simulink model "MultirotorSimPx4v1_8TuningRateCont"  (R2018b)
settings: Solver=VariableStepAuto  StartTime=0.0  StopTime=Simulation.T_END  MaxStep=Simulation.TS_MAX  RelTol=1e-3  EnableMultiTasking=on
PreLoadFcn:
  | % InitializeParameters;
undefined symbols (not defined in the file): DiscIntNeverNeededParam, Initial, Simulation, Uav, Wind
libraries: QuaternionLibrary x10, simulink x3, simulink_extras x2
(part 1 of 2)
settings Model: PauseTimes=0.99  Creator=jban039  LastModifiedBy=jban039
settings DataIOCC: Decimation=10  ExternalInput=getinputstruct(op1(2))  InitialState=getstatestruct(op)  SaveFormat=StructureWithTime  ReturnWorkspaceOutputs=on  OutputTimes=Simulation.T_OUT
settings OptimizationCC: LifeSpan=inf
settings DebuggingCC: ReadBeforeWriteMsg=DisableAll  WriteAfterWriteMsg=DisableAll  WriteAfterReadMsg=DisableAll  MultiTaskDSMMsg=none  UnconnectedLineMsg=none  AllowSymbolicDim=off  SFUnexpectedBacktrackingDiag=warning  SFNoUnconditionalDefaultTransitionDiag=warning  SFExecutionAtInitializationDiag=none
settings ModelReferenceCC: UpdateModelReferenceTargets=IfOutOfDate  ModelReferenceMinAlgLoopOccurrences=on  PropagateSignalLabelsOutOfModel=off
settings SFSimCC: SFSimEcho=off  SimUseLocalCustomCode=off
settings RTWCC: RTWUseLocalCustomCode=off
settings CodeAppCC: StateflowObjectComments=on
settings GRTTargetCC: TargetLangStandard=C89/C90 (ANSI)
settings ConfigComp: CovMetricSettings=dw  CovHtmlReporting=on  CovSaveCumulativeToWorkspaceVar=on  CovSaveSingleToWorkspaceVar=on  CovExternalEMLEnable=off

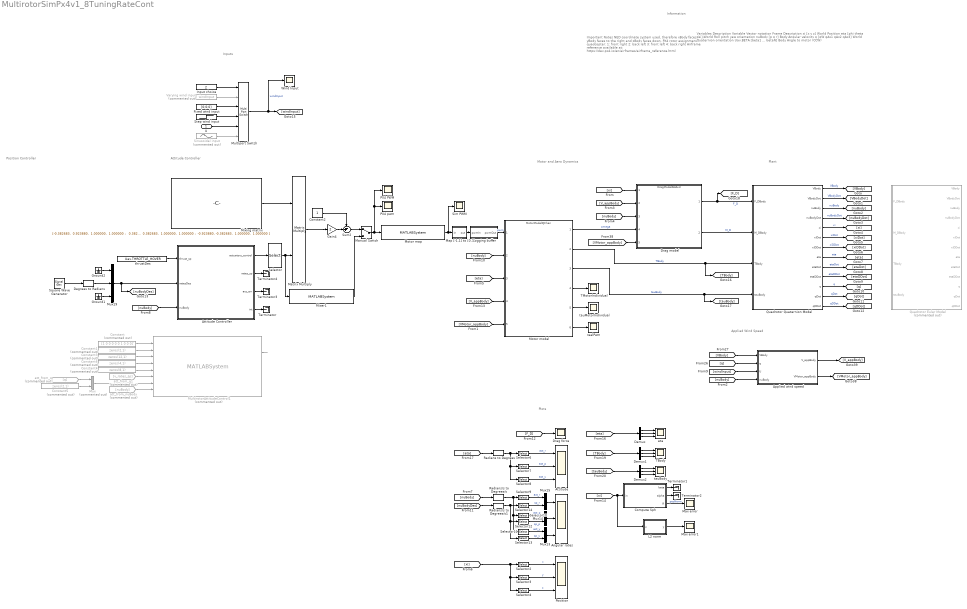
== system MultirotorSimPx4v1_8TuningRateCont ==
  note: Plots
  note: Inputs
  note: Motor and Aero Dynamics
  note: Plant
  note: Attitude Controller
  note: Position Controller
  note: Applied Wind Speed
  note: Important Notes
      |
      | NED coordinate system used, therefore xBody faces forward, yBody faces to the right and zBody faces down.
      | PX4 rotor assignment for quadcopter:
      | 1: front right
      | 2: back left
      | 3: front left
      | 4: back right
      | Airframe reference available at:
      | https://dev.px4.io/en/airframes/airframe_reference.html
  note: Variables Description
      |
      | Variable
      | Vector notation
      | Frame
      | Description
      |
      | xi
      | [x y z]
      | World
      | Position
      |
      | eta
      | [phi theta psi]
      | World
      | Roll pitch yaw orientation
      |
      | nuBody
      | [p q r]
      | Body
      | Angular velocity
      |
      | q
      | [qW qAx1 qAx2 qAx3]
      | World
      | Quaternion orientation
      |
      | Uav.BETA
      | [beta1 ... betaN]
      | Body
      | Angle to motor (CCW)
  note: Information
  U : Inport  PortDimensions=3
  Angular rates : Scope  NumInputPorts=3
  Applied wind speed : Subsystem
  Attitude : Scope  NumInputPorts=3
  Attitude Controller : Subsystem
  Compute Sph : MATLAB Function  TreatAsAtomicUnit=on
  Constant : Constant  Commented=on  Value=[1 0 0 0 0 0 1 0 0 0]'
  Constant1 : Constant  Commented=on  Value=zeros(2,1)
  Constant2 : Constant
  Constant3 : Constant  Commented=on  Value=zeros(12,1)
  Constant4 : Constant  Commented=on  Value=zeros(8,1)
  Constant5 : Constant  Commented=on  Value=zeros(2,1)
  Constant6 : Constant  Commented=on  Value=zeros(4,1)
  Degrees to Radians : simulink_extras/Transformations/Degrees to Radians
  Demux : Demux  Outputs=3
  Demux1 : Demux  Outputs=3
  Demux2 : Demux  Outputs=3
  Drag force : Scope
  Drag model : ModelReference  ModelNameDialog=DragModelAIAAv3  SimulationMode=Normal  ModelReferenceVersion=1.368
  Fixed wind input : Constant  Value=[0;0;0]
  Gain4 : Gain  Gain=2
  Ground1 : Ground
  Ground2 : Ground
  Input choice : Constant  Value=2
  L2 norm : MATLAB Function  TreatAsAtomicUnit=on
  Logging buffer : Subsystem
  Manual Switch : ManualSwitch
  Map [-1,1] to [0,1] : Subsystem
  Matrix Multiply : Product  Multiplication=Matrix(*)
  Max error : Scope
  Max error1 : Scope
  Mixer1 : MATLABSystem  System=MultirotorMixer  airframeConfig=6  useHorThrust=0  outputSatStatus=0  SimulateUsing=Code generation
      mask Type: MultirotorMixer
      mask Display:
      | disp(['MULTIROTOR' char(10) 'MIXER' char(10) 'octa_xneg']);
      | port_label('input',1,'actuatorsControl');
      | port_label('output',1,'px4PWM');
  Mixing matrix : Constant  Value=|
      | [-0.382683,  0.923880,  1.000000,  1.000000 ;
      |   0.382683, -0.923880,  1.000000,  1.000000 ;
      |  -0.923880,  0.382683, -1.000000,  1.000000 ;
      |  -0.382683, -0.923880, -1.000000,  1.000000 ;
      |   0.382683,  0.923880, -1.000000,  1.000000 ;
      |   0.923880, -0.382683, -1.000000,  1.000000 ;
      |   0.923880,  0.382683,  1.000000,  1.000000 ;
      |  -0.923880, -0.382683,  1.000000,  1.000000 ]
  Motor map : MATLABSystem  System=MotorMap  airframeConfig=5  SimulateUsing=Code generation
      mask Type: MotorMap
      mask Display:
      | disp(['MOTOR' char(10) 'MAP' char(10) 'octa_x']);
      | port_label('input',1,'px4PWM');
      | port_label('output',1,'simPWM');
  Motor model : ModelReference  ModelNameDialog=MotorModelZJChen  SimulationMode=Normal  ModelReferenceVersion=1.421
  Multiport Switch : MultiPortSwitch  Inputs=5
  MultirotorAttitudeControl1 : MATLABSystem  Commented=on  System=MulticopterAttitudeControl  acro_expo_rp=0.69  acro_expo_y=0.69  acro_pitch_max=720  acro_roll_max=720  acro_superexpo_rp=0.7  acro_superexpo_y=0.7  acro_yaw_max=540  airmode=0  d_term_cutoff_freq=30  pitch_rate_d=0.003  pitch_rate_ff=0  pitch_rate_i=0.05  pitch_rate_max=220  pitch_rate_p=0.15  pitch_p=6.5  pitch_rate_integ_lim=0.3  rattitude_thres=0.8  roll_rate_d=0.003  roll_rate_ff=0  roll_rate_i=0.05  roll_rate_max=220  roll_rate_p=0.15  roll_p=6.5  roll_rate_integ_lim=0.3  tpa_breakpoint_d=1  tpa_breakpoint_i=1  tpa_breakpoint_p=1  tpa_rate_d=0  tpa_rate_i=0  tpa_rate_p=0  yaw_rate_d=0  yaw_rate_ff=0  yaw_rate_i=0.1  yaw_rate_max=200  yaw_rate_p=0.2  yaw_auto_max=45  yaw_p=2.8  yaw_rate_integ_lim=0.3  man_throttle_min=0.08  man_tilt_max_deg=35  yaw_rate_scaling=200  throttle_hover=0.5  throttle_max=1  board_rotation_param=0  board_offset_x=0  board_offset_y=0  board_offset_z=0  bat_scale_en=0  throttle_curve=0  vehicle_status_is_rotary_wing=1  vehicle_status_is_vtol=0  loop_update_rate_hz=250  simple_mode=0  output_rates=1  SimulateUsing=Interpreted execution
      mask Type: MulticopterAttitudeControl
      mask Display:
      | disp(['MulticopterAttitudeControl' char(10) '' char(10) 'v1.82']);
      | port_label('input',1,'v_control_mode_flags');
      | port_label('input',2,'vehicle_land_detected');
      | port_label('input',3,'saturation_status');
      | port_label('input',4,'manual_control_sp');
      | port_label('input',5,'v_att_sp');
      | port_label('input',6,'v_rates_sp');
      | port_label('input',7,'v_att_in');
      | port_label('input',8,'sensor_gyro');
      | port_label('output',1,'actuatorsControl');
      | port_label('output',2,'attRateSp');
  Mux : Mux  Commented=on  Inputs=2
  Mux13 : Mux  Inputs=2
  Mux14 : Mux  Inputs=2
  Mux15 : Mux  Inputs=2
  Mux19 : Mux  Inputs=3
  PX4 PWM : Scope
  PX4 pwm : Scope
  Position : Scope  NumInputPorts=3
  Quadrotor Euler Model : Subsystem  Commented=on
  Quadrotor Quaternion Model : Subsystem
  "Radians to Degrees " : QuaternionLibrary/Radians to Degrees   SystemSampleTime=-1
  Radians/s to Degrees/s : QuaternionLibrary/Radians//s to Degrees//s  SystemSampleTime=-1
  Radians/s to Degrees/s1 : QuaternionLibrary/Radians//s to Degrees//s  SystemSampleTime=-1
  Selector : Selector  InputPortWidth=8  IndexOptions=Index vector (dialog)  Indices=[1:4]  OutputSizes=1
  Selector{3,7,10,12} (4 alike) : Selector  InputPortWidth=3  IndexOptions=Index vector (dialog)  Indices=2  OutputSizes=1
  Selector{4,8,11,13} (4 alike) : Selector  InputPortWidth=3  IndexOptions=Index vector (dialog)  Indices=3  OutputSizes=1
  Selector{2,6,9,14} (4 alike) : Selector  InputPortWidth=3  IndexOptions=Index vector (dialog)  Indices=1  OutputSizes=1
  Sim PWM : Scope
  Sinusoidal input : Sin  Commented=on  Amplitude=Wind.Ampl  Bias=Wind.Bias  Frequency=Wind.Freq  SampleTime=0
  Square Wave Generator : SignalGenerator  WaveForm=square  Amplitude=50  Frequency=2
  Step wind input : Step  Time=5  Before=[3 0 0]'  After=[5 0 0]'  SampleTime=0
  Sum2 : Sum  Inputs=-+|
  TBody : Scope  NumInputPorts=3
  TMotorIndividual : Scope
  Terminator{,1..4} (5 alike) : Terminator
  Varying wind input : FromWorkspace  Commented=on  VariableName=windInput  SampleTime=0
  Wind Input : Scope
  att_from_nuBody : From  Commented=on  GotoTag=nuBody
  att_from_q : From  Tag=q  Commented=on  GotoTag=q
  att_from_q1 : From  Tag=q  Commented=on  GotoTag=v_rates_sp
  eta : Scope  NumInputPorts=3
  realPwm : Scope
  tauBody : Scope  NumInputPorts=3
  tauMotorIndividual : Scope
  thrustDes : Constant  Value=Uav.THROTTLE_HOVER
  wires:
  Motor model/1 -> Drag model/4  "omega"
  Motor model/2 -> Quadrotor Quaternion Model/3(TBody), [TBody]  "TBody"
  Drag model/2 -> Quadrotor Quaternion Model/2(M_DBody)  "M_D"
  Quadrotor Quaternion Model/1(VBody) -> [VBody]  "VBody"
  Quadrotor Quaternion Model/2(VBodyDot) -> [VBodyDot]  "VBodyDot"
  Quadrotor Quaternion Model/3(nuBody) -> [nuBody]  "nuBody"
  Quadrotor Quaternion Model/4(nuBodyDot) -> [nuBodyDot]  "nuBodyDot"
  Quadrotor Quaternion Model/5(xi) -> [xi]  "xi"
  Quadrotor Quaternion Model/6(xiDot) -> [xiDot]  "xiDot"
  Quadrotor Quaternion Model/7(xiDDot) -> [xiDDot]  "xiDDot"
  Quadrotor Quaternion Model/8(eta) -> [eta]  "eta"
  Quadrotor Quaternion Model/9(etaDot) -> [etaDot]  "etaDot"
  Quadrotor Quaternion Model/10(etaDDot) -> [etaDDot]  "etaDDot"
  [V_appBody] -> Drag model/2
  [nuBody] -> Motor model/2
  Quadrotor Quaternion Model/11(q) -> [q]  "q"
  Quadrotor Quaternion Model/12(qDot) -> [qDot]  "qDot"
  Quadrotor Quaternion Model/13(qDDot) -> [qDDot]  "qDDot"
  Drag model/1 -> Quadrotor Quaternion Model/1(F_DBody), [F_D]  "F_D"
  Logging buffer/1(pwmOut) -> Motor model/1  "pwm"
  Manual Switch/1 -> PX4 PWM/1, PX4 pwm/1, Motor map/1
  [nuBody] -> Drag model/3
  [eta] -> Motor model/3
  [V_appBody] -> Motor model/4
  Motor model/4 -> TMotorIndividual/1
  Motor model/5 -> tauMotorIndividual/1
  [xi] -> Drag model/1
  [VMotor_appBody] -> Motor model/5
  [VMotor_appBody] -> Drag model/5
  Motor model/3 -> Quadrotor Quaternion Model/4(tauBody), [tauBody]  "tauBody"
  [VBody] -> Applied wind speed/1(VBody)
  [q] -> Applied wind speed/2(q)
  [windInput] -> Applied wind speed/3(U)
  Applied wind speed/1(V_appBody) -> [V_appBody]
  Applied wind speed/2(VMotor_appBody) -> [VMotor_appBody]
  [nuBody] -> Applied wind speed/4(nuBody)
  Motor model/6 -> realPwm/1
  [nuBody] -> Attitude Controller/3(nuBody)
  Motor map/1 -> Sim PWM/1, Map [-1,1] to [0,1]/1(in)
  Map [-1,1] to [0,1]/1(out) -> Logging buffer/1(pwmIn)
  Selector/1 -> Matrix Multiply/2, Mixer1/1
  Mixing matrix/1 -> Matrix Multiply/1
  Attitude Controller/1(actuators_control) -> Selector/1
  Gain4/1 -> Sum2/2
  Constant2/1 -> Sum2/1
  Attitude Controller/4(int) -> Terminator/1
  [xi] -> L2 norm/1(u), Compute Sph/1(in)
  [eta] -> Demux/1
  Demux/1 -> eta/1
  Demux/2 -> eta/2
  Demux/3 -> eta/3
  [eta] -> "Radians to Degrees "/1
  "Radians to Degrees "/1 -> Selector6/1, Selector7/1, Selector8/1
  Selector8/1 -> Attitude/3  "act_y"
  Selector7/1 -> Attitude/2  "act_p"
  Selector6/1 -> Attitude/1  "act_r"
  Varying wind input/1 -> Multiport Switch/2
  Fixed wind input/1 -> Multiport Switch/3
  Multiport Switch/1 -> Wind Input/1, [windInput]  "windInput"
  Demux1/3 -> TBody/3
  Demux1/2 -> TBody/2
  [TBody] -> Demux1/1
  Demux1/1 -> TBody/1
  Demux2/1 -> tauBody/1
  [tauBody] -> Demux2/1
  Demux2/2 -> tauBody/2
  Demux2/3 -> tauBody/3
  Step wind input/1 -> Multiport Switch/4
  Input choice/1 -> Multiport Switch/1
  Mux19/1 -> Attitude Controller/2(ratesDes), [nuBodyDes]
  Matrix Multiply/1 -> Gain4/1
  Compute Sph/1(beta) -> Terminator1/1
  Compute Sph/2(alpha) -> Terminator2/1
  Compute Sph/3(R) -> Max error/1  "posNorm"
  U/1 -> Multiport Switch/5
  [F_D] -> Drag force/1
  Sinusoidal input/1 -> Multiport Switch/6
  L2 norm/1(y) -> Max error1/1
  Square Wave Generator/1 -> Degrees to Radians/1
  Degrees to Radians/1 -> Mux19/2
  Ground2/1 -> Mux19/1
  Ground1/1 -> Mux19/3
  thrustDes/1 -> Attitude Controller/1(thrust_sp)
  [nuBodyDes] -> Radians/s to Degrees/s1/1
  Selector13/1 -> Mux13/2  "sp_y"
  Selector12/1 -> Mux14/2  "sp_p"
  Selector14/1 -> Mux15/2  "sp_r"
  Radians/s to Degrees/s1/1 -> Selector12/1, Selector13/1, Selector14/1
  Mux13/1 -> Angular rates/3
  [nuBody] -> Radians/s to Degrees/s/1
  Radians/s to Degrees/s/1 -> Selector10/1, Selector11/1, Selector9/1
  Mux14/1 -> Angular rates/2
  Mux15/1 -> Angular rates/1
  Selector11/1 -> Mux13/1  "act_y"
  Selector10/1 -> Mux14/1  "act_p"
  Selector9/1 -> Mux15/1  "act_r"
  att_from_q1/1 -> MultirotorAttitudeControl1/6
  Constant6/1 -> MultirotorAttitudeControl1/4
  Mux/1 -> MultirotorAttitudeControl1/7
  Constant5/1 -> Mux/2
  Constant4/1 -> MultirotorAttitudeControl1/5
  Constant3/1 -> MultirotorAttitudeControl1/3
  Constant1/1 -> MultirotorAttitudeControl1/2
  Constant/1 -> MultirotorAttitudeControl1/1
  att_from_nuBody/1 -> MultirotorAttitudeControl1/8
  att_from_q/1 -> Mux/1
  MultirotorAttitudeControl1/1 -> ?
  Attitude Controller/3(acc_err) -> Terminator3/1
  Attitude Controller/2(rates_sp) -> Terminator4/1
  Mixer1/1 -> Manual Switch/2
  Selector4/1 -> Position/3  "z"
  [xi] -> Selector2/1, Selector3/1, Selector4/1
  Selector3/1 -> Position/2  "y"
  Selector2/1 -> Position/1  "x"
  Sum2/1 -> Manual Switch/1

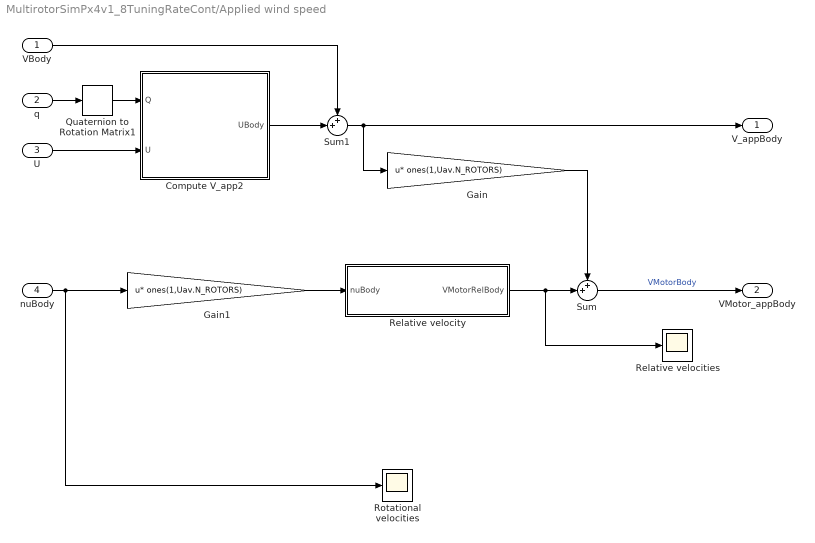
== system MultirotorSimPx4v1_8TuningRateCont/Applied wind speed ==
  VBody : Inport  Unit=m/s
  q : Inport  Port=2
  U : Inport  Port=3  Unit=m/s
  nuBody : Inport  Port=4  Unit=rad/s
  Compute V_app2 : MATLAB Function  TreatAsAtomicUnit=on
  Gain : Gain  Gain=ones(1,Uav.N_ROTORS)  Multiplication=Matrix(u*K)
  Gain1 : Gain  Gain=ones(1,Uav.N_ROTORS)  Multiplication=Matrix(u*K)
  Quaternion to Rotation Matrix1 : QuaternionLibrary/Quaternion to Rotation Matrix
  Relative velocities : Scope
  Relative velocity : MATLAB Function  TreatAsAtomicUnit=on
  Rotational velocities : Scope
  Sum : Sum  Inputs=++|
  Sum1 : Sum  Inputs=++|
  V_appBody : Outport  Unit=m/s
  VMotor_appBody : Outport  Port=2  Unit=m/s  PortDimensions=[3,Uav.N_ROTORS]
  wires:
  U/1 -> Compute V_app2/2(U)
  Sum/1 -> VMotor_appBody/1  "VMotorBody"
  Quaternion to Rotation Matrix1/1 -> Compute V_app2/1(Q)
  nuBody/1 -> Gain1/1, Rotational velocities/1
  Gain/1 -> Sum/1
  VBody/1 -> Sum1/1
  q/1 -> Quaternion to Rotation Matrix1/1
  Relative velocity/1(VMotorRelBody) -> Relative velocities/1, Sum/2
  Compute V_app2/1(UBody) -> Sum1/2
  Sum1/1 -> Gain/1, V_appBody/1
  Gain1/1 -> Relative velocity/1(nuBody)

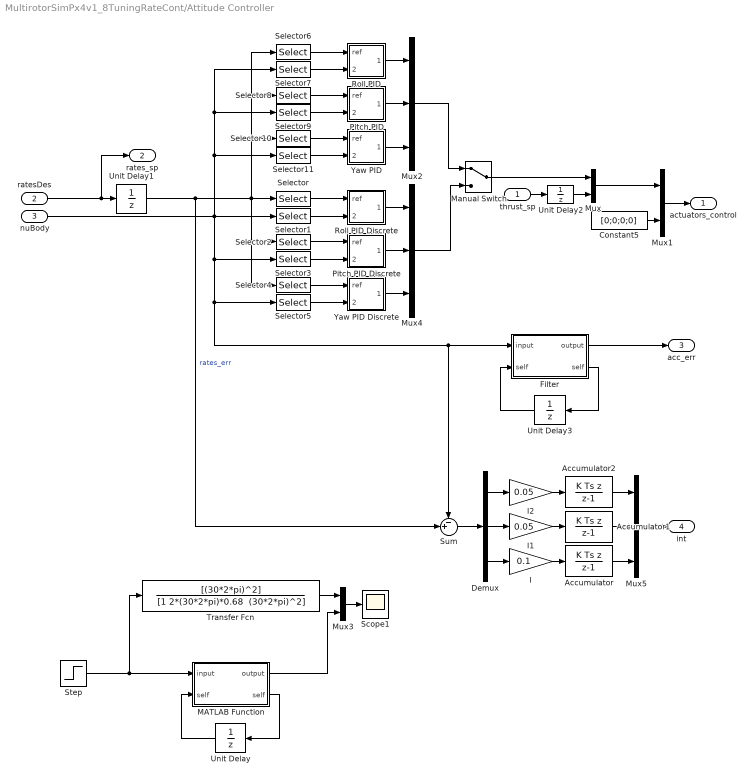
== system MultirotorSimPx4v1_8TuningRateCont/Attitude Controller ==
  thrust_sp : Inport  PortDimensions=1
  ratesDes : Inport  Port=2  SampleTime=1/250
  nuBody : Inport  Port=3  SampleTime=1/250
  Accumulator : DiscreteIntegrator  IntegratorMethod=Integration: Backward Euler  SampleTime=1/250  LimitOutput=on  UpperSaturationLimit=0.3  LowerSaturationLimit=-0.3  ICPrevOutput=DiscIntNeverNeededParam  ICPrevScaledInput=DiscIntNeverNeededParam
  Accumulator1 : DiscreteIntegrator  IntegratorMethod=Integration: Backward Euler  SampleTime=1/250  LimitOutput=on  UpperSaturationLimit=0.3  LowerSaturationLimit=-0.3  ICPrevOutput=DiscIntNeverNeededParam  ICPrevScaledInput=DiscIntNeverNeededParam
  Accumulator2 : DiscreteIntegrator  IntegratorMethod=Integration: Backward Euler  SampleTime=1/250  LimitOutput=on  UpperSaturationLimit=0.3  LowerSaturationLimit=-0.3  ICPrevOutput=DiscIntNeverNeededParam  ICPrevScaledInput=DiscIntNeverNeededParam
  Constant5 : Constant  Value=[0;0;0;0]
  Demux : Demux  Outputs=3
  Filter : MATLAB Function  TreatAsAtomicUnit=on  SystemSampleTime=1/250
  I : Gain  Gain=0.1
  I1 : Gain  Gain=0.05
  I2 : Gain  Gain=0.05
  MATLAB Function : MATLAB Function  TreatAsAtomicUnit=on  SystemSampleTime=1/250
  Manual Switch : ManualSwitch
  Mux : Mux  Inputs=2
  Mux1 : Mux  Inputs=2
  Mux2 : Mux  Inputs=3
  Mux3 : Mux  Inputs=2
  Mux4 : Mux  Inputs=3
  Mux5 : Mux  Inputs=3
  Pitch PID : Subsystem
      mask Display: disp('PID(s)')
  Pitch PID Discrete : Subsystem
      mask Display: disp('PID(s)')
  Roll PID : Subsystem
      mask Display: disp('PID(s)')
  Roll PID Discrete : Subsystem
      mask Display: disp('PID(s)')
  Scope1 : Scope
  Selector{,1,6..7} (4 alike) : Selector  InputPortWidth=3  IndexOptions=Index vector (dialog)  Indices=1  OutputSizes=1
  Selector{4..5,10..11} (4 alike) : Selector  InputPortWidth=3  IndexOptions=Index vector (dialog)  Indices=3  OutputSizes=1
  Selector{2..3,8..9} (4 alike) : Selector  InputPortWidth=3  IndexOptions=Index vector (dialog)  Indices=2  OutputSizes=1
  Step : Step  Time=0.5  SampleTime=0
  Sum : Sum  Inputs=-+|
  Transfer Fcn : TransferFcn  Numerator=[(30*2*pi)^2]  Denominator="[1 2*(30*2*pi)*0.68  (30*2*pi)^2]"
  Unit Delay : UnitDelay  InitialCondition=zeros(13,1)  SampleTime=1/250
  Unit Delay1 : UnitDelay  SampleTime=1/250
  Unit Delay2 : UnitDelay  SampleTime=1/250
  Unit Delay3 : UnitDelay  InitialCondition=zeros(13,1)  SampleTime=1/250
  Yaw PID : Subsystem
      mask Display: disp('PID(s)')
  Yaw PID Discrete : Subsystem
      mask Display: disp('PID(s)')
  actuators_control : Outport  PortDimensions=8
  rates_sp : Outport  Port=2
  acc_err : Outport  Port=3  PortDimensions=3
  int : Outport  Port=4  PortDimensions=3
  wires:
  Sum/1 -> Demux/1
  Mux5/1 -> int/1
  Demux/3 -> I/1
  Demux/2 -> I1/1
  Demux/1 -> I2/1
  Accumulator/1 -> Mux5/3
  Accumulator1/1 -> Mux5/2
  Accumulator2/1 -> Mux5/1
  I2/1 -> Accumulator2/1
  I1/1 -> Accumulator1/1
  I/1 -> Accumulator/1
  Selector9/1 -> Pitch PID/2(meas)
  Selector11/1 -> Yaw PID/2(meas)
  Selector10/1 -> Yaw PID/1(ref)
  Selector8/1 -> Pitch PID/1(ref)
  Selector7/1 -> Roll PID/2(meas)
  Selector6/1 -> Roll PID/1(ref)
  Selector5/1 -> Yaw PID Discrete/2(mes)
  Selector3/1 -> Pitch PID Discrete/2(mes)
  Selector1/1 -> Roll PID Discrete/2(mes)
  Filter/1(output) -> acc_err/1
  Filter/2(self) -> Unit Delay3/1
  Unit Delay3/1 -> Filter/2("self ")
  Mux4/1 -> Manual Switch/2
  thrust_sp/1 -> Unit Delay2/1
  Mux2/1 -> Manual Switch/1
  Selector/1 -> Roll PID Discrete/1(ref)
  Selector2/1 -> Pitch PID Discrete/1(ref)
  Selector4/1 -> Yaw PID Discrete/1(ref)
  Yaw PID Discrete/1(Out) -> Mux4/3
  Roll PID Discrete/1(Out) -> Mux4/1
  Pitch PID Discrete/1(Out) -> Mux4/2
  Transfer Fcn/1 -> Mux3/1
  Mux3/1 -> Scope1/1
  MATLAB Function/1(output) -> Mux3/2
  Step/1 -> Transfer Fcn/1, MATLAB Function/1(input)
  Unit Delay/1 -> MATLAB Function/2("self ")
  MATLAB Function/2(self) -> Unit Delay/1
  Pitch PID/1(Out) -> Mux2/2
  Roll PID/1(Out) -> Mux2/1
  Yaw PID/1(Out) -> Mux2/3
  nuBody/1 -> Selector1/1, Selector3/1, Selector5/1, Filter/1(input), Sum/1, Selector7/1, Selector9/1, Selector11/1
  Mux/1 -> Mux1/1
  Constant5/1 -> Mux1/2
  Mux1/1 -> actuators_control/1
  ratesDes/1 -> Unit Delay1/1, rates_sp/1
  Unit Delay2/1 -> Mux/2
  Unit Delay1/1 -> Selector4/1, Selector2/1, Selector/1, Selector6/1, Selector8/1, Selector10/1, Sum/2  "rates_err"
  Manual Switch/1 -> Mux/1

== system MultirotorSimPx4v1_8TuningRateCont/Logging buffer ==
  pwmIn : Inport
  Rate Transition : RateTransition  Commented=through  SCDEnableBlockLinearizationSpecification=on
  pwmOut : Outport
  wires:
  pwmIn/1 -> Rate Transition/1
  Rate Transition/1 -> pwmOut/1

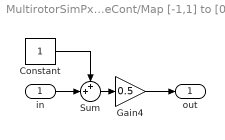
== system MultirotorSimPx4v1_8TuningRateCont/Map [-1,1] to [0,1] ==
  in : Inport
  Constant : Constant
  Gain4 : Gain  Gain=0.5
  Sum : Sum  Inputs=++|
  out : Outport
  wires:
  Sum/1 -> Gain4/1
  Gain4/1 -> out/1
  in/1 -> Sum/2
  Constant/1 -> Sum/1

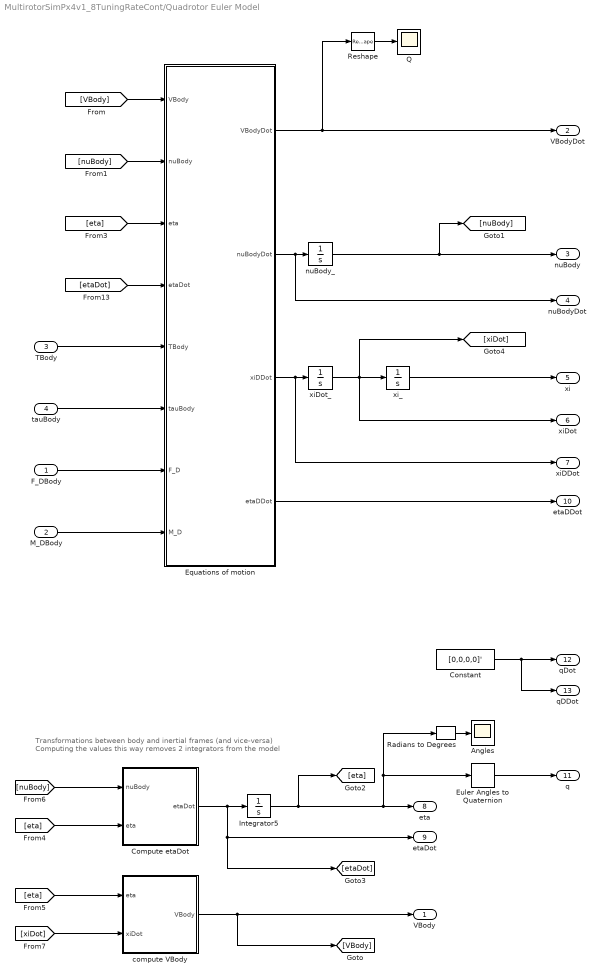
== system MultirotorSimPx4v1_8TuningRateCont/Quadrotor Euler Model ==
  note: Transformations between body and inertial frames (and vice-versa)
      | Computing the values this way removes 2 integrators from the model
  F_DBody : Inport  Unit=N
  M_DBody : Inport  Port=2  Unit=N*m
  TBody : Inport  Port=3  Unit=N
  tauBody : Inport  Port=4  Unit=N*m
  Angles : Scope
  Compute etaDot : MATLAB Function  TreatAsAtomicUnit=on
  Constant : Constant  Value=[0,0,0,0]'
  Equations of motion : MATLAB Function  TreatAsAtomicUnit=on
  Euler Angles to Quaternion : QuaternionLibrary/Euler Angles to Quaternion
  Integrator5 : Integrator  InitialCondition=Initial.ETA  ContinuousStateAttributes='eta'
  Q : Scope
  Radians to Degrees : simulink_extras/Transformations/Radians to Degrees
  Reshape : Reshape  OutputDimensionality=Column vector (2-D)
  compute VBody : MATLAB Function  TreatAsAtomicUnit=on
  nuBody_ : Integrator  InitialCondition=Initial.NU_BODY  ContinuousStateAttributes='nuBody'
  xiDot_ : Integrator  InitialCondition=Initial.XI_DOT  ContinuousStateAttributes='xiDot'
  xi_ : Integrator  InitialCondition=Initial.XI  ContinuousStateAttributes='xi'
  VBody : Outport  Unit=m/s
  VBodyDot : Outport  Port=2  Unit=m/s^2
  nuBody : Outport  Port=3  Unit=rad/s
  nuBodyDot : Outport  Port=4  Unit=rad/s^2
  xi : Outport  Port=5  Unit=m
  xiDot : Outport  Port=6  Unit=m/s
  xiDDot : Outport  Port=7  Unit=m/s^2
  eta : Outport  Port=8  Unit=rad
  etaDot : Outport  Port=9  Unit=rad/s
  etaDDot : Outport  Port=10  Unit=rad/s^2
  q : Outport  Port=11
  qDot : Outport  Port=12
  qDDot : Outport  Port=13
  wires:
  Radians to Degrees/1 -> Angles/1
  Constant/1 -> qDot/1, qDDot/1
  Euler Angles to Quaternion/1 -> q/1
  Integrator5/1 -> [eta], eta/1, Euler Angles to Quaternion/1, Radians to Degrees/1
  Compute etaDot/1(etaDot) -> Integrator5/1, [etaDot], etaDot/1
  [eta] -> Compute etaDot/2(eta)
  compute VBody/1(VBody) -> [VBody], VBody/1
  [eta] -> compute VBody/1(eta)
  [nuBody] -> Compute etaDot/1(nuBody)
  [xiDot] -> compute VBody/2(xiDot)
  [etaDot] -> Equations of motion/4(etaDot)
  xiDot_/1 -> xiDot/1, [xiDot], xi_/1
  Reshape/1 -> Q/1
  Equations of motion/4(etaDDot) -> etaDDot/1
  [eta] -> Equations of motion/3(eta)
  Equations of motion/2(nuBodyDot) -> nuBodyDot/1, nuBody_/1
  nuBody_/1 -> nuBody/1, [nuBody]
  M_DBody/1 -> Equations of motion/8(M_D)
  F_DBody/1 -> Equations of motion/7(F_D)
  Equations of motion/3(xiDDot) -> xiDDot/1, xiDot_/1
  TBody/1 -> Equations of motion/5(TBody)
  tauBody/1 -> Equations of motion/6(tauBody)
  [VBody] -> Equations of motion/1(VBody)
  [nuBody] -> Equations of motion/2(nuBody)
  xi_/1 -> xi/1
  Equations of motion/1(VBodyDot) -> VBodyDot/1, Reshape/1

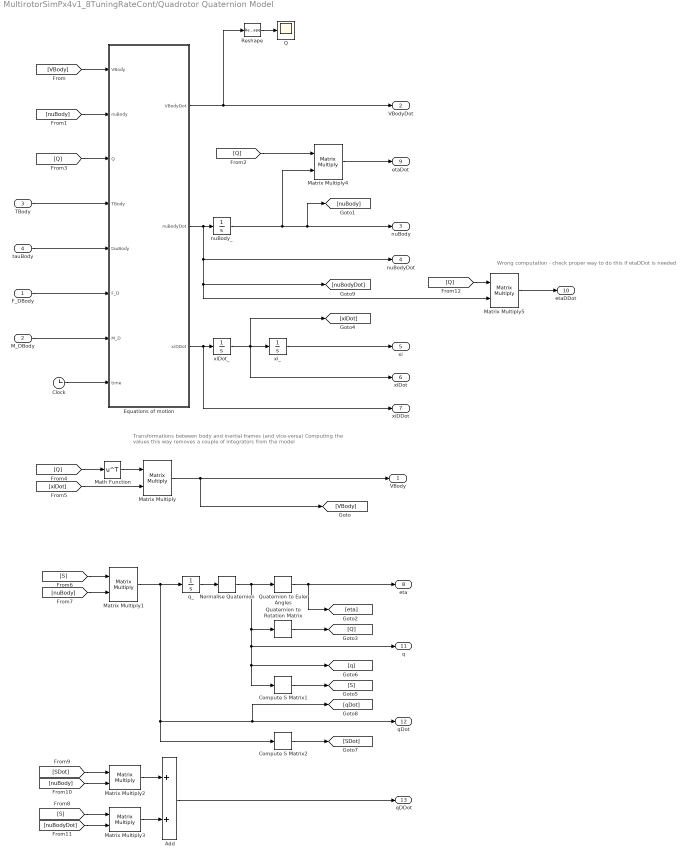
== system MultirotorSimPx4v1_8TuningRateCont/Quadrotor Quaternion Model ==
  note: Transformations between body and inertial frames (and vice-versa)
      | Computing the values this way removes a couple of integrators from the model
  note: Wrong computation - check proper way to do this if etaDDot is needed
  F_DBody : Inport  Unit=N
  M_DBody : Inport  Port=2  Unit=N*m
  TBody : Inport  Port=3  Unit=N
  tauBody : Inport  Port=4  Unit=N*m
  Add : Sum
  Clock : Clock
  Compute S Matrix1 : QuaternionLibrary/Compute S Matrix
  Compute S Matrix2 : QuaternionLibrary/Compute S Matrix
  Equations of motion : MATLAB Function  TreatAsAtomicUnit=on
  Math Function : Math  Operator=transpose  SaturateOnIntegerOverflow=on
  Matrix Multiply{,1..5} (6 alike) : Product  Multiplication=Matrix(*)
  Normalise Quaternion : QuaternionLibrary/Normalise Quaternion
  Q : Scope
  Quaternion to Euler Angles : QuaternionLibrary/Quaternion to Euler Angles
  Quaternion to Rotation Matrix : QuaternionLibrary/Quaternion to Rotation Matrix
  Reshape : Reshape  OutputDimensionality=Column vector (2-D)
  nuBody_ : Integrator  InitialCondition=Initial.NU_BODY  ContinuousStateAttributes='nuBody'
  q_ : Integrator  InitialCondition=Initial.Q  ContinuousStateAttributes='q'
  xiDot_ : Integrator  InitialCondition=Initial.XI_DOT  ContinuousStateAttributes='xiDot'
  xi_ : Integrator  InitialCondition=Initial.XI  ContinuousStateAttributes='xi'
  VBody : Outport  Unit=m/s
  VBodyDot : Outport  Port=2  Unit=m/s^2
  nuBody : Outport  Port=3  Unit=rad/s
  nuBodyDot : Outport  Port=4  Unit=rad/s^2
  xi : Outport  Port=5  Unit=m
  xiDot : Outport  Port=6  Unit=m/s
  xiDDot : Outport  Port=7  Unit=m/s^2
  eta : Outport  Port=8  Unit=rad
  etaDot : Outport  Port=9  Unit=rad/s
  etaDDot : Outport  Port=10  Unit=rad/s^2
  q : Outport  Port=11
  qDot : Outport  Port=12
  qDDot : Outport  Port=13
  wires:
  Clock/1 -> Equations of motion/8(time)
  xiDot_/1 -> xiDot/1, [xiDot], xi_/1
  Reshape/1 -> Q/1
  Matrix Multiply5/1 -> etaDDot/1
  [Q] -> Matrix Multiply5/1
  Add/1 -> qDDot/1
  [Q] -> Matrix Multiply4/1
  Compute S Matrix1/1 -> [S]
  Normalise Quaternion/1 -> Quaternion to Rotation Matrix/1, [q], Compute S Matrix1/1, q/1, Quaternion to Euler Angles/1
  Matrix Multiply3/1 -> Add/2
  Matrix Multiply2/1 -> Add/1
  [nuBodyDot] -> Matrix Multiply3/2
  [nuBody] -> Matrix Multiply2/2
  [SDot] -> Matrix Multiply2/1
  Matrix Multiply1/1 -> q_/1, Compute S Matrix2/1, [qDot], qDot/1
  [S] -> Matrix Multiply3/1
  Compute S Matrix2/1 -> [SDot]
  [nuBody] -> Matrix Multiply1/2
  [S] -> Matrix Multiply1/1
  Math Function/1 -> Matrix Multiply/1
  [xiDot] -> Matrix Multiply/2
  [Q] -> Math Function/1
  [Q] -> Equations of motion/3(Q)
  Quaternion to Rotation Matrix/1 -> [Q]
  Matrix Multiply4/1 -> etaDot/1
  Quaternion to Euler Angles/1 -> [eta], eta/1
  q_/1 -> Normalise Quaternion/1
  Equations of motion/2(nuBodyDot) -> [nuBodyDot], Matrix Multiply5/2, nuBodyDot/1, nuBody_/1
  nuBody_/1 -> nuBody/1, [nuBody], Matrix Multiply4/2
  M_DBody/1 -> Equations of motion/7(M_D)
  Matrix Multiply/1 -> [VBody], VBody/1
  F_DBody/1 -> Equations of motion/6(F_D)
  Equations of motion/3(xiDDot) -> xiDDot/1, xiDot_/1
  TBody/1 -> Equations of motion/4(TBody)
  tauBody/1 -> Equations of motion/5(tauBody)
  [VBody] -> Equations of motion/1(VBody)
  [nuBody] -> Equations of motion/2(nuBody)
  xi_/1 -> xi/1
  Equations of motion/1(VBodyDot) -> VBodyDot/1, Reshape/1

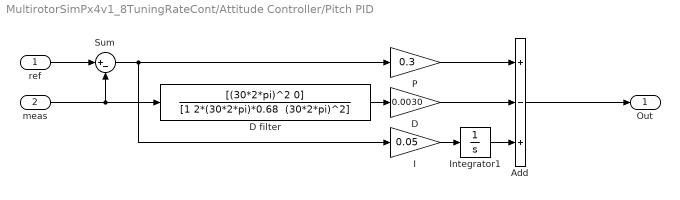
== system MultirotorSimPx4v1_8TuningRateCont/Attitude Controller/Pitch PID ==
  ref : Inport
  meas : Inport  Port=2
  Add : Sum  Inputs=+-+
  D : Gain  Gain=0.0030
  D filter : TransferFcn  Numerator=[(30*2*pi)^2 0]  Denominator="[1 2*(30*2*pi)*0.68  (30*2*pi)^2]"
  I : Gain  Gain=0.05
  Integrator1 : Integrator  LimitOutput=on  UpperSaturationLimit=0.3  LowerSaturationLimit=-0.3
  P : Gain  Gain=0.3
  Sum : Sum  Inputs=|+-
  Out : Outport
  wires:
  Add/1 -> Out/1
  P/1 -> Add/1
  Integrator1/1 -> Add/3
  D filter/1 -> D/1
  Sum/1 -> I/1, P/1
  D/1 -> Add/2
  I/1 -> Integrator1/1
  ref/1 -> Sum/1
  meas/1 -> D filter/1, Sum/2

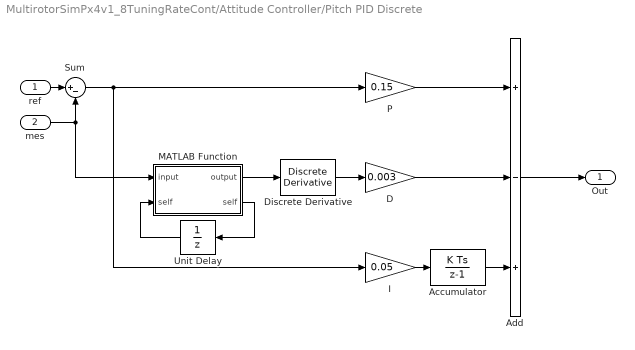
== system MultirotorSimPx4v1_8TuningRateCont/Attitude Controller/Pitch PID Discrete ==
  ref : Inport  SampleTime=1/250
  mes : Inport  Port=2  SampleTime=1/250
  Accumulator : DiscreteIntegrator  SampleTime=1/250  LimitOutput=on  UpperSaturationLimit=0.3  LowerSaturationLimit=-0.3  ICPrevOutput=DiscIntNeverNeededParam  ICPrevScaledInput=DiscIntNeverNeededParam
  Add : Sum  Inputs=+-+
  D : Gain  Gain=0.003
  Discrete Derivative : simulink/Discrete/Discrete Derivative  gainval=1.0  ICPrevScaledInput=0.0  OutMin=[]  OutMax=[]  OutDataType=fixdt(1, 16)  OutScaling=2^-10  DoSatur=off
  I : Gain  Gain=0.05
  MATLAB Function : MATLAB Function  TreatAsAtomicUnit=on  SystemSampleTime=1/250
  P : Gain  Gain=0.15
  Sum : Sum  Inputs=|+-
  Unit Delay : UnitDelay  InitialCondition=zeros(9,1)  SampleTime=1/250
  Out : Outport  SampleTime=1/250
  wires:
  Sum/1 -> I/1, P/1
  Unit Delay/1 -> MATLAB Function/2("self ")
  MATLAB Function/2(self) -> Unit Delay/1
  I/1 -> Accumulator/1
  D/1 -> Add/2
  MATLAB Function/1(output) -> Discrete Derivative/1
  Accumulator/1 -> Add/3
  P/1 -> Add/1
  Add/1 -> Out/1
  Discrete Derivative/1 -> D/1
  ref/1 -> Sum/1
  mes/1 -> MATLAB Function/1(input), Sum/2

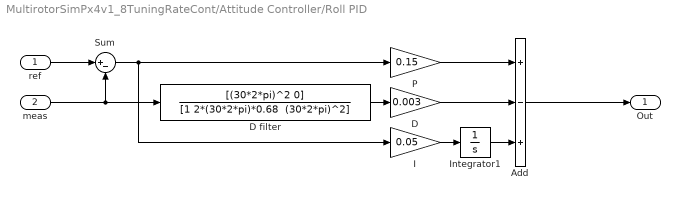
== system MultirotorSimPx4v1_8TuningRateCont/Attitude Controller/Roll PID ==
  ref : Inport
  meas : Inport  Port=2
  Add : Sum  Inputs=+-+
  D : Gain  Gain=0.003
  D filter : TransferFcn  Numerator=[(30*2*pi)^2 0]  Denominator="[1 2*(30*2*pi)*0.68  (30*2*pi)^2]"
  I : Gain  Gain=0.05
  Integrator1 : Integrator  LimitOutput=on  UpperSaturationLimit=0.3  LowerSaturationLimit=-0.3
  P : Gain  Gain=0.15
  Sum : Sum  Inputs=|+-
  Out : Outport
  wires:
  meas/1 -> Sum/2, D filter/1
  ref/1 -> Sum/1
  I/1 -> Integrator1/1
  D/1 -> Add/2
  Sum/1 -> P/1, I/1
  D filter/1 -> D/1
  Integrator1/1 -> Add/3
  P/1 -> Add/1
  Add/1 -> Out/1

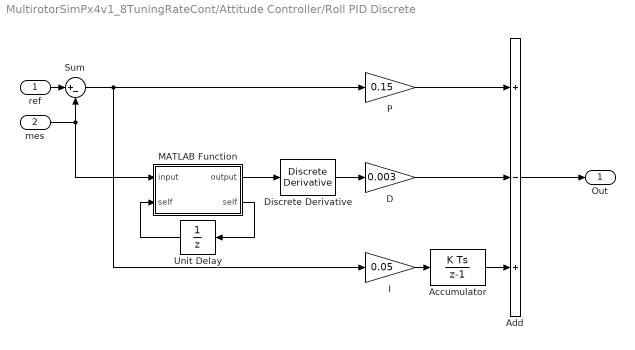
== system MultirotorSimPx4v1_8TuningRateCont/Attitude Controller/Roll PID Discrete ==
  ref : Inport  SampleTime=1/250
  mes : Inport  Port=2  SampleTime=1/250
  Accumulator : DiscreteIntegrator  SampleTime=1/250  LimitOutput=on  UpperSaturationLimit=0.3  LowerSaturationLimit=-0.3  ICPrevOutput=DiscIntNeverNeededParam  ICPrevScaledInput=DiscIntNeverNeededParam
  Add : Sum  Inputs=+-+
  D : Gain  Gain=0.003
  Discrete Derivative : simulink/Discrete/Discrete Derivative  gainval=1.0  ICPrevScaledInput=0.0  OutMin=[]  OutMax=[]  OutDataType=fixdt(1, 16)  OutScaling=2^-10  DoSatur=off
  I : Gain  Gain=0.05
  MATLAB Function : MATLAB Function  TreatAsAtomicUnit=on  SystemSampleTime=1/250
  P : Gain  Gain=0.15
  Sum : Sum  Inputs=|+-
  Unit Delay : UnitDelay  InitialCondition=zeros(9,1)  SampleTime=1/250
  Out : Outport  SampleTime=1/250
  wires:
  mes/1 -> Sum/2, MATLAB Function/1(input)
  ref/1 -> Sum/1
  Discrete Derivative/1 -> D/1
  Add/1 -> Out/1
  P/1 -> Add/1
  Accumulator/1 -> Add/3
  MATLAB Function/1(output) -> Discrete Derivative/1
  D/1 -> Add/2
  I/1 -> Accumulator/1
  MATLAB Function/2(self) -> Unit Delay/1
  Unit Delay/1 -> MATLAB Function/2("self ")
  Sum/1 -> P/1, I/1

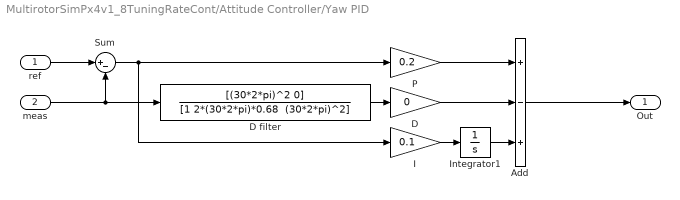
== system MultirotorSimPx4v1_8TuningRateCont/Attitude Controller/Yaw PID ==
  ref : Inport
  meas : Inport  Port=2
  Add : Sum  Inputs=+-+
  D : Gain  Gain=0
  D filter : TransferFcn  Numerator=[(30*2*pi)^2 0]  Denominator="[1 2*(30*2*pi)*0.68  (30*2*pi)^2]"
  I : Gain  Gain=0.1
  Integrator1 : Integrator  LimitOutput=on  UpperSaturationLimit=0.3  LowerSaturationLimit=-0.3
  P : Gain  Gain=0.2
  Sum : Sum  Inputs=|+-
  Out : Outport
  wires:
  meas/1 -> Sum/2, D filter/1
  ref/1 -> Sum/1
  I/1 -> Integrator1/1
  D/1 -> Add/2
  Sum/1 -> P/1, I/1
  D filter/1 -> D/1
  Integrator1/1 -> Add/3
  P/1 -> Add/1
  Add/1 -> Out/1

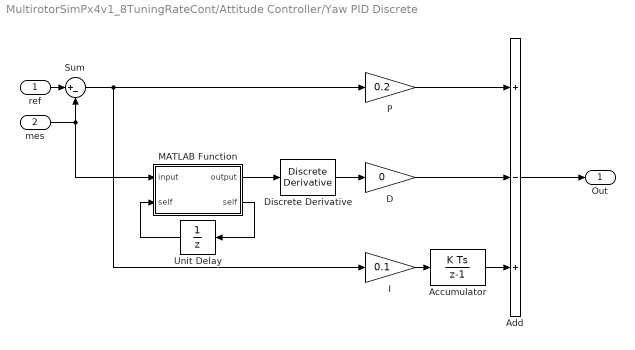
== system MultirotorSimPx4v1_8TuningRateCont/Attitude Controller/Yaw PID Discrete ==
  ref : Inport  SampleTime=1/250
  mes : Inport  Port=2  SampleTime=1/250
  Accumulator : DiscreteIntegrator  SampleTime=1/250  LimitOutput=on  UpperSaturationLimit=0.3  LowerSaturationLimit=-0.3  ICPrevOutput=DiscIntNeverNeededParam  ICPrevScaledInput=DiscIntNeverNeededParam
  Add : Sum  Inputs=+-+
  D : Gain  Gain=0
  Discrete Derivative : simulink/Discrete/Discrete Derivative  gainval=1.0  ICPrevScaledInput=0.0  OutMin=[]  OutMax=[]  OutDataType=fixdt(1, 16)  OutScaling=2^-10  DoSatur=off
  I : Gain  Gain=0.1
  MATLAB Function : MATLAB Function  TreatAsAtomicUnit=on  SystemSampleTime=1/250
  P : Gain  Gain=0.2
  Sum : Sum  Inputs=|+-
  Unit Delay : UnitDelay  InitialCondition=zeros(9,1)  SampleTime=1/250
  Out : Outport  SampleTime=1/250
  wires:
  mes/1 -> Sum/2, MATLAB Function/1(input)
  ref/1 -> Sum/1
  Discrete Derivative/1 -> D/1
  Add/1 -> Out/1
  P/1 -> Add/1
  Accumulator/1 -> Add/3
  MATLAB Function/1(output) -> Discrete Derivative/1
  D/1 -> Add/2
  I/1 -> Accumulator/1
  MATLAB Function/2(self) -> Unit Delay/1
  Unit Delay/1 -> MATLAB Function/2("self ")
  Sum/1 -> P/1, I/1

== matlab function MultirotorSimPx4v1_8TuningRateCont/Quadrotor Euler Model/Equations of motion ==
  data: VBody input; VBodyDot output; nuBody input; eta input; etaDot input; TBody input size=3; tauBody input size=3; F_D input size=3; M_D input size=3; nuBodyDot output; Uav parameter; xiDDot output; etaDDot output
function [VBodyDot, nuBodyDot, xiDDot, etaDDot] = QuadrotorQuaternionModel(...
    VBody, nuBody, eta, etaDot, TBody, tauBody, F_D, M_D, Uav )
%#codegen

%% Rotation matrices
% Precompute sines and cosines
sPhi   = sin(eta(1));
sTheta = sin(eta(2));
sPsi   = sin(eta(3));
cPhi   = cos(eta(1));
cTheta = cos(eta(2));
cPsi   = cos(eta(3));
tTheta = tan(eta(2));

phiDot   = etaDot(1);
thetaDot = etaDot(2);

% Body frame to inertial frame
R = [cPsi*cTheta, cPsi*sTheta*sPhi-sPsi*cPhi, cPsi*sTheta*cPhi+sPsi*sPhi;
     sPsi*cTheta, sPsi*sTheta*sPhi+cPsi*cPhi, sPsi*sTheta*cPhi-cPsi*sPhi;
     -sTheta,     cTheta*sPhi,                cTheta*cPhi+sPsi*sPhi];

WInvertDot = [...
    0,  phiDot*cPhi*tTheta+thetaDot*sPhi/cTheta^2,    -phiDot*sPhi*cTheta+thetaDot*cPhi/cTheta^2;
    0, -phiDot*sPhi,                                  -phiDot*cPhi;
	0,  phiDot*cPhi/cTheta+phiDot*sPhi*tTheta/cTheta, -phiDot*sPhi/cTheta+thetaDot*cPhi*tTheta/cTheta];

WInvert = [1, sPhi*tTheta,  cPhi*tTheta;
           0, cPhi,        -sPhi;
           0, sPhi/cTheta,  cPhi/cTheta];


%% Moments and Forces
% Body frame accelerations
VBodyDot  = (1/Uav.M) * (R'*Uav.G + TBody - cross(nuBody, Uav.M*VBody) + F_D);
nuBodyDot = Uav.I \ (tauBody - cross(nuBody, Uav.I*nuBody) + M_D);

% Inertial frame accelerations
xiDDot = (1/Uav.M)*(Uav.G + R*TBody + R*F_D);
etaDDot = WInvertDot*nuBody + WInvert*nuBodyDot;

end

== matlab function MultirotorSimPx4v1_8TuningRateCont/Applied wind speed/Relative velocity ==
  data: nuBody input; Uav parameter; VMotorRelBody output
function VMotorRelBody = relativeMotorVelocity( nuBody , Uav )
%#codegen
    VMotorRelBody = cross( nuBody, Uav.L_VEC );
end

== matlab function MultirotorSimPx4v1_8TuningRateCont/Applied wind speed/Compute V_app2 ==
  data: Q input; UBody output; U input size=3
function UBody = computeUBody(Q, U)
%#codegen

% Rotation matrix from Wind frame to Inertial frame
% Wind frame SEU, inertial frame NED
R_U = [1,  0, 0;
       0, -1, 0;
       0,  0, 1];
   
UBody = Q' * R_U * U;

== matlab function MultirotorSimPx4v1_8TuningRateCont/Attitude Controller/Filter ==
  data: input input; self input; output output; self output
function [ output, self ] = Filter( input, self )
    % 'Decode' self vector
    obj.lp_filters_d_a1 = self(1);
    obj.lp_filters_d_a2 = self(2);
    obj.lp_filters_d_b0 = self(3);
    obj.lp_filters_d_b1 = self(4);
    obj.lp_filters_d_b2 = self(5);
    obj.lp_filters_d_cutoff_freq = 30;
    obj.lp_filters_d_delay_element_1 = self(7:9);
    obj.lp_filters_d_delay_element_2 = self(10:12);
    init = self(13);
    
    % Variables
    sample_freq = 250;
    cutoff_freq = 30;
    
    if ~init
        obj = LowPassFilter2pVectorSetCutOffFrequency( obj, sample_freq, cutoff_freq );
        init = 1;
    end
    
    [obj, output] = LowPassFilter2pVector3Apply( obj, input );

    % 'Encode' self vector
    self(1)     = obj.lp_filters_d_a1;
    self(2)     = obj.lp_filters_d_a2;
    self(3)     = obj.lp_filters_d_b0;
    self(4)     = obj.lp_filters_d_b1;
    self(5)     = obj.lp_filters_d_b2;
    self(6)     = obj.lp_filters_d_cutoff_freq;
    self(7:9)    = obj.lp_filters_d_delay_element_1;
    self(10:12) = obj.lp_filters_d_delay_element_2;
    self(13) = init;
end

function [obj, output] = LowPassFilter2pVector3Apply( obj, sample )
    %LOWPASSFILTER2PVECTOR3APPLY Apply low pass filter
    %   Based on code from PX4 Firmware:
    %       https://github.com/PX4/Firmware/blob/master/src/lib/mathlib/math/filter/LowPassFilter2pVector3f.hpp
    %   Written:       J.X.J. Bannwarth, 2019/01/16
    %   Last modified: J.X.J. Bannwarth, 2019/01/21
    delay_element_0 = sample - obj.lp_filters_d_delay_element_1.*obj.lp_filters_d_a1 - obj.lp_filters_d_delay_element_2.*obj.lp_filters_d_a2;
    output = delay_element_0.*obj.lp_filters_d_b0 + obj.lp_filters_d_delay_element_1.*obj.lp_filters_d_b1 + obj.lp_filters_d_delay_element_2*obj.lp_filters_d_b2;
    obj.lp_filters_d_delay_element_2 = obj.lp_filters_d_delay_element_1;
    obj.lp_filters_d_delay_element_1 = delay_element_0;
end

    function obj =  LowPassFilter2pVectorSetCutOffFrequency( obj, sample_freq, cutoff_freq )
    %LOWPASSFILTER2PVECTOR3SETCUTOFFFREQUENCY Set cutoff frequency
    %   Based on code from PX4 Firmware:
    %       https://github.com/PX4/Firmware/blob/master/src/lib/mathlib/math/filter/LowPassFilter2pVector3f.cpp
    %   Written:       J.X.J. Bannwarth, 2019/01/16
    %   Last modified: J.X.J. Bannwarth, 2019/01/21
    obj.lp_filters_d_cutoff_freq = cutoff_freq;

    % Reset delay elements on filter change
    obj.lp_filters_d_delay_element_1 = zeros(3,1);
    obj.lp_filters_d_delay_element_2 = zeros(3,1);

    if (obj.lp_filters_d_cutoff_freq <= 0.0)
        % No filtering
        obj.lp_filters_d_b0 = 1.0;
        obj.lp_filters_d_b1 = 0.0;
        obj.lp_filters_d_b2 = 0.0;

        obj.lp_filters_d_a1 = 0.0;
        obj.lp_filters_d_a2 = 0.0;
        return
    end

    fr = sample_freq / obj.lp_filters_d_cutoff_freq;
    ohm = tan( pi / fr);
    c = 1.0 + 2.0 * cos( pi / 4.0) * ohm + ohm * ohm;

    obj.lp_filters_d_b0 = ohm * ohm / c;
    obj.lp_filters_d_b1 = 2.0 * obj.lp_filters_d_b0;
    obj.lp_filters_d_b2 = obj.lp_filters_d_b0;

    obj.lp_filters_d_a1 = 2.0 * (ohm * ohm - 1.0) / c;
    obj.lp_filters_d_a2 = (1.0 - 2.0 * cos(pi / 4.0) * ohm + ohm * ohm) / c;
end

% function output = LowPassFilter2pVectorReset( obj, sample )
%     %LOWPASSFILTER2PVECTOR3SETCUTOFFFREQUENCY Set cutoff frequency
%     %   Based on code from PX4 Firmware:
%     %       https://github.com/PX4/Firmware/blob/master/src/lib/mathlib/math/filter/LowPassFilter2pVector3f.cpp
%     %   Written:       J.X.J. Bannwarth, 2019/01/16
%     %   Last modified: J.X.J. Bannwarth, 2019/01/21
%     dval = sample ./ (obj.lp_filters_d_b0 + obj.lp_filters_d_b1 + obj.lp_filters_d_b2);
% 
%     if (isfinite( dval(1) ) && isfinite( dval(2) ) && isfinite( dval(3) ))
%         obj.lp_filters_d_delay_element_1 = dval;
%         obj.lp_filters_d_delay_element_2 = dval;
%     else
%         obj.lp_filters_d_delay_element_1 = sample;
%         obj.lp_filters_d_delay_element_2 = sample;
%     end
% 
%     output = LowPassFilter2pVector3Apply( obj, sample );
% end

== matlab function MultirotorSimPx4v1_8TuningRateCont/Attitude Controller/MATLAB Function ==
  data: input input; self input; output output; self output
function [ output, self ] = Filter( input, self )
    % 'Decode' self vector
    obj.lp_filters_d_a1 = self(1);
    obj.lp_filters_d_a2 = self(2);
    obj.lp_filters_d_b0 = self(3);
    obj.lp_filters_d_b1 = self(4);
    obj.lp_filters_d_b2 = self(5);
    obj.lp_filters_d_cutoff_freq = self(6);
    obj.lp_filters_d_delay_element_1 = self(7:9);
    obj.lp_filters_d_delay_element_2 = self(10:12);
    init = self(13);
    
    % Variables
    sample_freq = 250;
    cutoff_freq = 30;
    
    if ~init
        obj = LowPassFilter2pVectorSetCutOffFrequency( obj, sample_freq, cutoff_freq );
        init = 1;
    end
    
    [obj, output] = LowPassFilter2pVector3Apply( obj, input );

    % 'Encode' self vector
    self(1)     = obj.lp_filters_d_a1;
    self(2)     = obj.lp_filters_d_a2;
    self(3)     = obj.lp_filters_d_b0;
    self(4)     = obj.lp_filters_d_b1;
    self(5)     = obj.lp_filters_d_b2;
    self(6)     = obj.lp_filters_d_cutoff_freq;
    self(7:9)    = obj.lp_filters_d_delay_element_1;
    self(10:12) = obj.lp_filters_d_delay_element_2;
    self(13) = init;
end

function [obj, output] = LowPassFilter2pVector3Apply( obj, sample )
    %LOWPASSFILTER2PVECTOR3APPLY Apply low pass filter
    %   Based on code from PX4 Firmware:
    %       https://github.com/PX4/Firmware/blob/master/src/lib/mathlib/math/filter/LowPassFilter2pVector3f.hpp
    %   Written:       J.X.J. Bannwarth, 2019/01/16
    %   Last modified: J.X.J. Bannwarth, 2019/01/21
    delay_element_0 = sample - obj.lp_filters_d_delay_element_1.*obj.lp_filters_d_a1 - obj.lp_filters_d_delay_element_2.*obj.lp_filters_d_a2;
    output = delay_element_0.*obj.lp_filters_d_b0 + obj.lp_filters_d_delay_element_1.*obj.lp_filters_d_b1 + obj.lp_filters_d_delay_element_2*obj.lp_filters_d_b2;
    obj.lp_filters_d_delay_element_2 = obj.lp_filters_d_delay_element_1;
    obj.lp_filters_d_delay_element_1 = delay_element_0;
end

    function obj =  LowPassFilter2pVectorSetCutOffFrequency( obj, sample_freq, cutoff_freq )
    %LOWPASSFILTER2PVECTOR3SETCUTOFFFREQUENCY Set cutoff frequency
    %   Based on code from PX4 Firmware:
    %       https://github.com/PX4/Firmware/blob/master/src/lib/mathlib/math/filter/LowPassFilter2pVector3f.cpp
    %   Written:       J.X.J. Bannwarth, 2019/01/16
    %   Last modified: J.X.J. Bannwarth, 2019/01/21
    obj.lp_filters_d_cutoff_freq = cutoff_freq;

    % Reset delay elements on filter change
    obj.lp_filters_d_delay_element_1 = zeros(3,1);
    obj.lp_filters_d_delay_element_2 = zeros(3,1);

    if (obj.lp_filters_d_cutoff_freq <= 0.0)
        % No filtering
        obj.lp_filters_d_b0 = 1.0;
        obj.lp_filters_d_b1 = 0.0;
        obj.lp_filters_d_b2 = 0.0;

        obj.lp_filters_d_a1 = 0.0;
        obj.lp_filters_d_a2 = 0.0;
        return
    end

    fr = sample_freq / obj.lp_filters_d_cutoff_freq;
    ohm = tan( pi / fr);
    c = 1.0 + 2.0 * cos( pi / 4.0) * ohm + ohm * ohm;

    obj.lp_filters_d_b0 = ohm * ohm / c;
    obj.lp_filters_d_b1 = 2.0 * obj.lp_filters_d_b0;
    obj.lp_filters_d_b2 = obj.lp_filters_d_b0;

    obj.lp_filters_d_a1 = 2.0 * (ohm * ohm - 1.0) / c;
    obj.lp_filters_d_a2 = (1.0 - 2.0 * cos(pi / 4.0) * ohm + ohm * ohm) / c;
end

% function output = LowPassFilter2pVectorReset( obj, sample )
%     %LOWPASSFILTER2PVECTOR3SETCUTOFFFREQUENCY Set cutoff frequency
%     %   Based on code from PX4 Firmware:
%     %       https://github.com/PX4/Firmware/blob/master/src/lib/mathlib/math/filter/LowPassFilter2pVector3f.cpp
%     %   Written:       J.X.J. Bannwarth, 2019/01/16
%     %   Last modified: J.X.J. Bannwarth, 2019/01/21
%     dval = sample ./ (obj.lp_filters_d_b0 + obj.lp_filters_d_b1 + obj.lp_filters_d_b2);
% 
%     if (isfinite( dval(1) ) && isfinite( dval(2) ) && isfinite( dval(3) ))
%         obj.lp_filters_d_delay_element_1 = dval;
%         obj.lp_filters_d_delay_element_2 = dval;
%     else
%         obj.lp_filters_d_delay_element_1 = sample;
%         obj.lp_filters_d_delay_element_2 = sample;
%     end
% 
%     output = LowPassFilter2pVector3Apply( obj, sample );
% end

== matlab function MultirotorSimPx4v1_8TuningRateCont/Compute Sph ==
  data: in input; beta output; alpha output; R output
function [beta, alpha, R] = computeSph(in)
%#codegen

% Convert from polar to spherical coordinates
[ beta, alpha, R ] = cart2sph( in(1), in(2), in(3) );

== matlab function MultirotorSimPx4v1_8TuningRateCont/Quadrotor Euler Model/Compute etaDot ==
  data: nuBody input; eta input; etaDot output
function etaDot = computeEtaDot(nuBody, eta)
%#codegen

sPhi = sin(eta(1));
cPhi = cos(eta(1));
cTheta = cos(eta(2));
tTheta = tan(eta(2));
      
WInverse = [1, sPhi*tTheta,  cPhi*tTheta;
            0, cPhi,        -sPhi;
            0, sPhi/cTheta,  cPhi/cTheta];

etaDot = WInverse*nuBody;

== matlab function MultirotorSimPx4v1_8TuningRateCont/Attitude Controller/Pitch PID Discrete/MATLAB Function ==
  data: input input; self input; output output; self output
function [ output, self ] = Filter( input, self )
    % 'Decode' self vector
    obj.lp_filters_d_a1 = self(1);
    obj.lp_filters_d_a2 = self(2);
    obj.lp_filters_d_b0 = self(3);
    obj.lp_filters_d_b1 = self(4);
    obj.lp_filters_d_b2 = self(5);
    obj.lp_filters_d_cutoff_freq = self(6);
    obj.lp_filters_d_delay_element_1 = self(7);
    obj.lp_filters_d_delay_element_2 = self(8);
    init = self(9);
    
    % Variables
    sample_freq = 250;
    cutoff_freq = 30;
    
    if ~init
        obj = LowPassFilter2pVectorSetCutOffFrequency( obj, sample_freq, cutoff_freq );
        init = 1;
    end
    
    [obj, output] = LowPassFilter2pVector3Apply( obj, input );

    % 'Encode' self vector
    self(1)     = obj.lp_filters_d_a1;
    self(2)     = obj.lp_filters_d_a2;
    self(3)     = obj.lp_filters_d_b0;
    self(4)     = obj.lp_filters_d_b1;
    self(5)     = obj.lp_filters_d_b2;
    self(6)     = obj.lp_filters_d_cutoff_freq;
    self(7)    = obj.lp_filters_d_delay_element_1;
    self(8) = obj.lp_filters_d_delay_element_2;
    self(9) = init;
end

function [obj, output] = LowPassFilter2pVector3Apply( obj, sample )
    %LOWPASSFILTER2PVECTOR3APPLY Apply low pass filter
    %   Based on code from PX4 Firmware:
    %       https://github.com/PX4/Firmware/blob/master/src/lib/mathlib/math/filter/LowPassFilter2pVector3f.hpp
    %   Written:       J.X.J. Bannwarth, 2019/01/16
    %   Last modified: J.X.J. Bannwarth, 2019/01/21
    delay_element_0 = sample - obj.lp_filters_d_delay_element_1.*obj.lp_filters_d_a1 - obj.lp_filters_d_delay_element_2.*obj.lp_filters_d_a2;
    output = delay_element_0.*obj.lp_filters_d_b0 + obj.lp_filters_d_delay_element_1.*obj.lp_filters_d_b1 + obj.lp_filters_d_delay_element_2*obj.lp_filters_d_b2;
    obj.lp_filters_d_delay_element_2 = obj.lp_filters_d_delay_element_1;
    obj.lp_filters_d_delay_element_1 = delay_element_0;
end

    function obj =  LowPassFilter2pVectorSetCutOffFrequency( obj, sample_freq, cutoff_freq )
    %LOWPASSFILTER2PVECTOR3SETCUTOFFFREQUENCY Set cutoff frequency
    %   Based on code from PX4 Firmware:
    %       https://github.com/PX4/Firmware/blob/master/src/lib/mathlib/math/filter/LowPassFilter2pVector3f.cpp
    %   Written:       J.X.J. Bannwarth, 2019/01/16
    %   Last modified: J.X.J. Bannwarth, 2019/01/21
    obj.lp_filters_d_cutoff_freq = cutoff_freq;

    % Reset delay elements on filter change
    obj.lp_filters_d_delay_element_1 = 0;
    obj.lp_filters_d_delay_element_2 = 0;

    if (obj.lp_filters_d_cutoff_freq <= 0.0)
        % No filtering
        obj.lp_filters_d_b0 = 1.0;
        obj.lp_filters_d_b1 = 0.0;
        obj.lp_filters_d_b2 = 0.0;

        obj.lp_filters_d_a1 = 0.0;
        obj.lp_filters_d_a2 = 0.0;
        return
    end

    fr = sample_freq / obj.lp_filters_d_cutoff_freq;
    ohm = tan( pi / fr);
    c = 1.0 + 2.0 * cos( pi / 4.0) * ohm + ohm * ohm;

    obj.lp_filters_d_b0 = ohm * ohm / c;
    obj.lp_filters_d_b1 = 2.0 * obj.lp_filters_d_b0;
    obj.lp_filters_d_b2 = obj.lp_filters_d_b0;

    obj.lp_filters_d_a1 = 2.0 * (ohm * ohm - 1.0) / c;
    obj.lp_filters_d_a2 = (1.0 - 2.0 * cos(pi / 4.0) * ohm + ohm * ohm) / c;
end

% function output = LowPassFilter2pVectorReset( obj, sample )
%     %LOWPASSFILTER2PVECTOR3SETCUTOFFFREQUENCY Set cutoff frequency
%     %   Based on code from PX4 Firmware:
%     %       https://github.com/PX4/Firmware/blob/master/src/lib/mathlib/math/filter/LowPassFilter2pVector3f.cpp
%     %   Written:       J.X.J. Bannwarth, 2019/01/16
%     %   Last modified: J.X.J. Bannwarth, 2019/01/21
%     dval = sample ./ (obj.lp_filters_d_b0 + obj.lp_filters_d_b1 + obj.lp_filters_d_b2);
% 
%     if (isfinite( dval(1) ) && isfinite( dval(2) ) && isfinite( dval(3) ))
%         obj.lp_filters_d_delay_element_1 = dval;
%         obj.lp_filters_d_delay_element_2 = dval;
%     else
%         obj.lp_filters_d_delay_element_1 = sample;
%         obj.lp_filters_d_delay_element_2 = sample;
%     end
% 
%     output = LowPassFilter2pVector3Apply( obj, sample );
% end

== matlab function MultirotorSimPx4v1_8TuningRateCont/Quadrotor Euler Model/compute VBody ==
  data: eta input; VBody output; xiDot input
function VBody = computeVBody(eta, xiDot)
%#codegen

sphi = sin(eta(1));
sTheta = sin(eta(2));
sPsi = sin(eta(3));
cPhi = cos(eta(1));
cTheta = cos(eta(2));
cPsi = cos(eta(3));

R = [ cPsi*cTheta, cPsi*sTheta*sphi-sPsi*cPhi, cPsi*sTheta*cPhi+sPsi*sphi;
	  sPsi*cTheta, sPsi*sTheta*sphi+cPsi*cPhi, sPsi*sTheta*cPhi-cPsi*sphi;
     -sTheta,      cTheta*sphi,                cTheta*cPhi+sPsi*sphi];

VBody = R'*xiDot;

== matlab function MultirotorSimPx4v1_8TuningRateCont/L2 norm ==
  data: u input; y output
function y = l2norm( u )
    y = sqrt( dot(u, u) );
end
